simulink model "Omnilink"  (R2017a)
settings: Solver=FixedStepDiscrete  StartTime=0.0  StopTime=inf  FixedStep=1e-3  RelTol=1e-3  EnableMultiTasking=on
libraries: simulink x1
settings Model: Creator=wasonj  LastModifiedBy=rish5
settings DataIOCC: LimitDataPoints=on  MaxDataPoints=10000  SaveFormat=Array  SignalLoggingSaveFormat=ModelDataLogs
settings OptimizationCC: ExpressionDepthLimit=2147483647  LifeSpan=inf
settings DebuggingCC: UnderspecifiedInitializationDetection=Classic  MergeDetectMultiDrivingBlocksExec=none  SolverPrmCheckMsg=warning  FcnCallInpInsideContextMsg=warning  StateNameClashWarn=warning  SFUnexpectedBacktrackingDiag=warning  SFNoUnconditionalDefaultTransitionDiag=warning  SFExecutionAtInitializationDiag=none
settings HardwareCC: ProdBitPerPointer=32  ProdBitPerSizeT=32  ProdBitPerPtrDiffT=32  ProdLargestAtomicFloat=None  ProdIntDivRoundTo=Undefined  ProdEndianess=Unspecified  ProdWordSize=32  ProdHWDeviceType=32-bit Generic
settings ModelReferenceCC: PropagateSignalLabelsOutOfModel=off
settings RTWCC: SystemTargetFile=catsdll.tlc  TemplateMakefile=catsdll_vc.tmf  Description=CATS DLL Real-Time Target
settings STFCustomTargetCC: ModelReferenceCompliant=off  GeneratePreprocessorConditionals=Disable all  MATLABClassNameForMDSCustomization=Simulink.SoftwareTarget.TargetSpecificTriggerConfigurationBase  SystemTargetFile=catsdll.tlc
settings ConfigComp: CovMetricSettings=dw  CovHtmlReporting=on  CovSaveCumulativeToWorkspaceVar=on  CovSaveSingleToWorkspaceVar=on  CovExternalEMLEnable=off

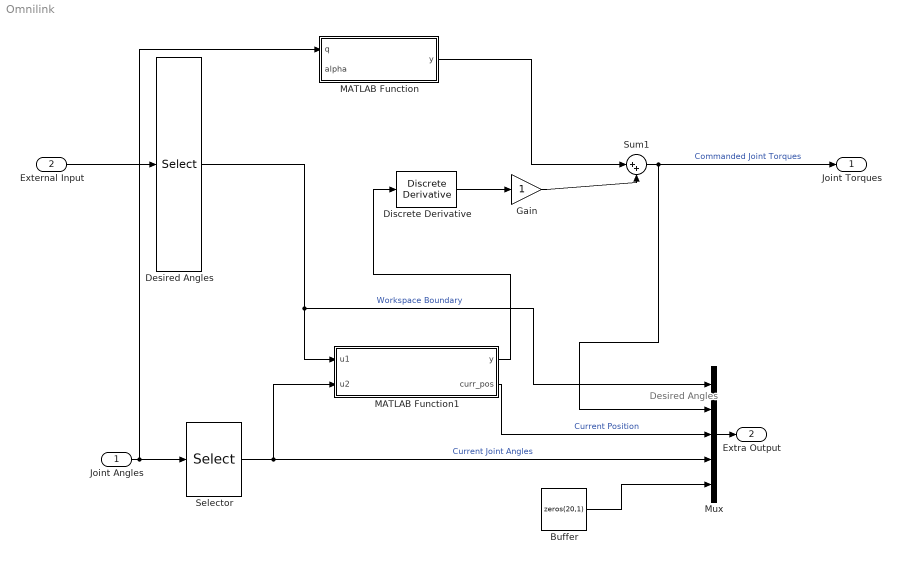
== system Omnilink ==
  note: Desired Angles
  Joint Angles : Inport  PortDimensions=6
  External Input : Inport  Port=2  PortDimensions=16
  Buffer : Constant  Value=zeros(20,1)
  Desired Angles : Selector  InputPortWidth=16  IndexOptions=Index vector (dialog)  Indices=[1:3]  OutputSizes=1
  Discrete Derivative : simulink/Discrete/Discrete Derivative  gainval=1.0  ICPrevScaledInput=0.0  InputProcessing=Inherited  OutMin=[]  OutMax=[]  OutDataType=fixdt(1, 16)  OutScaling=2^-10  DoSatur=off
  Gain : Gain
  MATLAB Function : MATLAB Function  TreatAsAtomicUnit=on
  MATLAB Function1 : MATLAB Function  TreatAsAtomicUnit=on
  Mux : Mux  Inputs=5
  Selector : Selector  InputPortWidth=6  IndexOptions=Index vector (dialog)  Indices=1:3  OutputSizes=1
  Sum1 : Sum  Inputs=|++
  Joint Torques : Outport  PortDimensions=3
  Extra Output : Outport  Port=2  PortDimensions=32
  wires:
  Joint Angles/1 -> Selector/1, MATLAB Function/1(q)
  Selector/1 -> MATLAB Function1/2(u2), Mux/4  "Current Joint Angles"
  Desired Angles/1 -> Mux/1, MATLAB Function1/1(u1)  "Workspace Boundary"
  Sum1/1 -> Joint Torques/1, Mux/2  "Commanded Joint Torques"
  Mux/1 -> Extra Output/1
  Buffer/1 -> Mux/5
  External Input/1 -> Desired Angles/1
  Discrete Derivative/1 -> Gain/1
  Gain/1 -> Sum1/2
  MATLAB Function/1(y) -> Sum1/1
  MATLAB Function1/2(curr_pos) -> Mux/3  "Current Position"
  MATLAB Function1/1(y) -> Discrete Derivative/1

== matlab function Omnilink/MATLAB Function1 ==
  data: y output; u1 input; curr_pos output; u2 input
function [y,curr_pos] = Haptic_Control(u1,u2)
des_pos = forward(u1(1),u1(2),u1(3)); %Based on other omni. In our project we need this to be based on camera sectioned image.

curr_pos = OmniForwardKinematics(u2(1),u2(2),u2(3)); %fwdkin to find current position

J = jacobian(u2(1),u2(2),u2(3)); %Jacobian using q_current as input

y = J'*(des_pos-curr_pos); %y is torque

y = sqrt(norm(y))*y/norm(y); %Scaling factor the other project used that we likely won't use

% Make haptic feedback like force-like spring, where repelling force = k*x
% k is stiffness of the spring, x is (desired_position based on image) - Forwardkin(q_current))
% torque = J'*F
% torque is the haptic feedback to the user
% Current challenge is how to define q_camera from sectioned image
%User should feel repulsion when they are in a "1" spot towards the nearest
%"0" spot. That force should increase as they go farther away from the
%nearest "0" spot. desired position is nearest "0" spot if in a "1"
%spot, else haptic torque is zero.
%Can't be based on user's direction in b/c that would require memory of
%user's pathway

% function [haptic_torque,curr_pos] = Feedback Controller(q,L)
% curr_pos = OmniForwardKinematics(q(1),q(2),q(3));
% if L = "1";
%     des_pos = nearest position where L = "0"
%     J = OmniJacobian(q(1),q(2),q(3));
%     k = 1; stiffness can be applied outside this function in simulink
%     haptic_torque = J'*k*(des_pos-curr_pos);
% else L = "0";
%     haptic_torque = J'*0;
% end

== matlab function Omnilink/MATLAB Function ==
  data: q input; y output; alpha input
function y = GravComp(q,alpha)
% Gravity Compensation
% Taken from previous Omni project
c2 = cos(q(2));
s2 = sin(q(2));
c3 = cos(q(3));
s3 = sin(q(3));
c4 = cos(q(4));
s4 = sin(q(4));
c5 = cos(q(5));
s5 = sin(q(5));
c6 = cos(q(6));
s6 = sin(q(6));
lambda = [0,0,0,0,0,0,0,0,0,0,0,0,0,0,0;...
-c2,0,-s2,-c2*c3+s2*s3,0,-c2*s3-c3*s2,...
-c2*c3+s3*s2,-c2*s3*s4-s2*c3*s4,-c2*s3*c4-s2*c3*c4,...
-c2*c3*c5+c2*s3*c4*c5+s2*s3*s5-s2*c3*c4*c5,...
-c2*s3*s4-s2*c3*s4,-c2*c3*s5-c2*s3*c4*c5+s2*s3*s5-s2*c3*c4*c5,...
-c2*c3*c5*c6+c2*s3*c4*s5*c6+s2*s3*c5*c6+s2*c3*c4*c5*c6,...
c2*c3*c5*s6-c2*s3*c4*s5*s6-c2*s3*s4*c6-s2*s3*c5*s6-s2*c3*c4*c5*s6-s2*c3*s4*c6,...
-c2*c3*s5-c2*s3*c4*c5+s2*s3*s5-s2*c3*c4*c5;...
0,0,0,s2*s3-c2*c3,0,-s2*c3-c2*s3,s2*s3-c2*c3,-s2*c3*s4-c2*s3*s4,-s2*c3*c4-c2*s3*c4,...
s2*s3*c5+s2*c3*c4*s5-c2*c3*c5+c2*s3*c4*s5,...
-s2*c3*s4-c2*s3*s4,s2*s3*s5-s2*c3*c4*c5-c2*c3*s5-c2*s3*c4*c5,...
s2*s3*c5*c6+s2*c3*c4*s5*c6-s2*c3*s4*s6-c2*c3*c5*c6+c2*s3*c4*s5*c6-c2*s3*s4*s6,...
-s2*s3*c5*s6-s2*c3*c4*s5*s6-s2*c3*s4*c6+c2*c3*c5*s6-c2*s3*c4*s5*s6-c2*s3*s4*c6,...
s2*s3*s5-s2*c3*c4*c5-c2*c3*s5-c2*s3*c4*c5];
y=lambda*alpha;
